simulink model "Copy_of_Simulink_demo_20240x2810x29"  (R2024a)
settings: Solver=ode4  StartTime=0.0  StopTime=200  FixedStep=1e-3  RelTol=1e-3
settings Model: Creator=20225074  LastModifiedBy=Leti
settings DebuggingCC: UnderSpecifiedDimensionMsg=warning

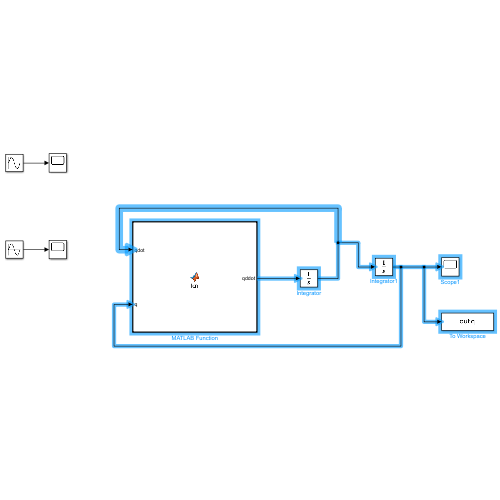
[thumbnail: Simulink's stored preview of the top-level diagram]
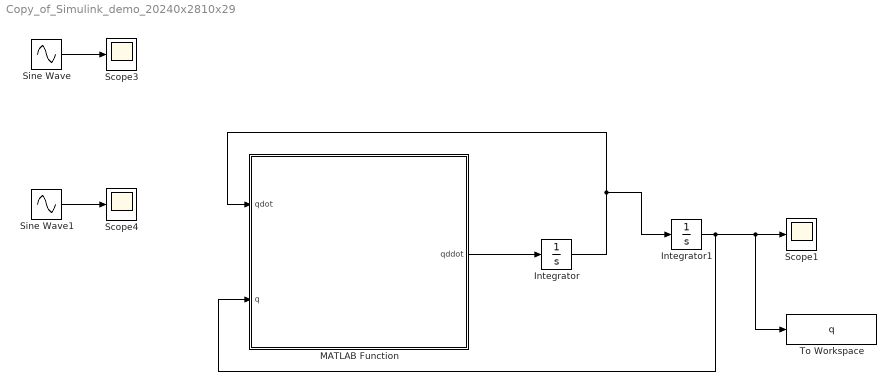
== system Copy_of_Simulink_demo_20240x2810x29 ==
  Integrator : Integrator  InitialCondition=[0;0]
  Integrator1 : Integrator  InitialCondition=[0;0.12]
  MATLAB Function : MATLAB Function  TreatAsAtomicUnit=on
  Scope1 : Scope
  Scope3 : Scope
  Scope4 : Scope
  Sine Wave : Sin  Amplitude=-4/5  Frequency=2  SampleTime=0
  Sine Wave1 : Sin  Amplitude=1/2  SampleTime=0
  To Workspace : ToWorkspace  VariableName=q  SampleTime=-1
  wires:
  MATLAB Function/1(qddot) -> Integrator/1
  Integrator/1 -> MATLAB Function/1(qdot), Integrator1/1
  Integrator1/1 -> Scope1/1, To Workspace/1, MATLAB Function/2(q)
  Sine Wave/1 -> Scope3/1
  Sine Wave1/1 -> Scope4/1

== matlab function Copy_of_Simulink_demo_20240x2810x29/MATLAB Function ==
  data: qdot input; q input; qddot output


function qddot = fcn(qdot,q)


% Variables

g = 9.81;
Lp = 0.5;
Lw = 1;
Mp = 1;
Mw = 0.2;
Jp = 0.083;
Jw = 0.1;
dphi = 0;
ktheta = 6.558;
dtheta = 0;
theta_ref = pi/2;
kphi = 0.114;
phi_ref = pi/2;


q1 = [q(1)-1.04762 ; q(2)-pi/2];


% Matrices

M = [Mp*Lp^2 + Mw*Lw^2 + Jp + Jw , Jw ; Jw , Jw];

D = [dtheta , 0 ; 0 , dphi];

K = [ktheta - 0.5*sqrt(3)*g*(Lp*Mp + Lw*Mw) , 0 ; 0 , kphi];

Kt = [0,0;0,0];

Ktot = K+Kt;

Qt = [0;0];

    
% Motion

qddot = (M \ (Qt - D * qdot - Ktot * q1));
